simulink model "ConverterDesign_R2015a"  (R2015a)
settings: Solver=FixedStepDiscrete  SolverMode=SingleTasking  StartTime=0.0  StopTime=15  FixedStep=10e-6  RelTol=1e-3
undefined symbols (not defined in the file): Ion, Lithium
libraries: powerlib x13, simulink x2, powerlib_meascontrol x2, electricdrivelib x1, re_lib x1
settings Model: CovMetricSettings=dwe  CovHtmlReporting=off  covSaveCumulativeToWorkspaceVar=off  CovSaveSingleToWorkspaceVar=off  CovExternalEMLEnable=on  Creator=debma  LastModifiedBy=debma
settings DataIOCC: LimitDataPoints=off  SaveFormat=Dataset  ReturnWorkspaceOutputs=on
settings DebuggingCC: SFUnexpectedBacktrackingDiag=error  SFNoUnconditionalDefaultTransitionDiag=error
settings HardwareCC: ProdBitPerPointer=64  ProdLargestAtomicFloat=Float  ProdIntDivRoundTo=Zero  ProdEndianess=LittleEndian  ProdHWDeviceType=Specified
settings ModelReferenceCC: PropagateSignalLabelsOutOfModel=on
settings SFSimCC: SimUseLocalCustomCode=on
settings RTWCC: RTWUseLocalCustomCode=on
settings GRTTargetCC: TargetLangStandard=C99 (ISO)
settings ConfigurationSet: Description=Simscape Multibody

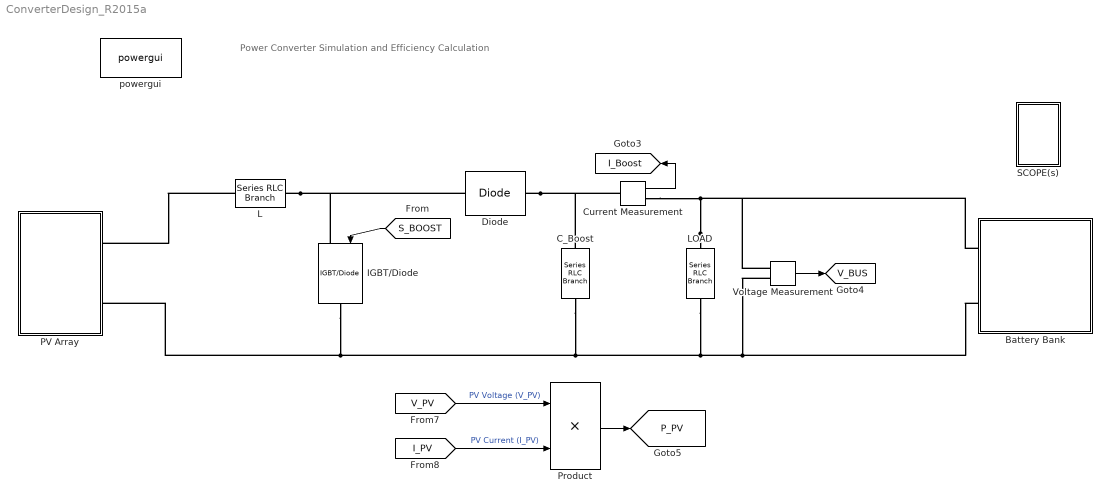
== system ConverterDesign_R2015a ==
  note: Power Converter Simulation and Efficiency Calculation
  Battery Bank : Subsystem
  C_Boost : powerlib/Elements/Series RLC Branch  LConnTagsString=__new0  RConnTagsString=__new0  BranchType=RC  Resistance=1e-4  Inductance=1e-3  SetiL0=off  InitialCurrent=0  Capacitance=3330e-6  Setx0=off  InitialVoltage=0  Measurements=None
  Current Measurement : powerlib/Measurements/Current Measurement  PhasorSimulation=off  OutputType=Complex  PSBequivalent=0
  Diode : powerlib/Power Electronics/Diode  Ron=0.001  Lon=0  Vf=0.8  IC=0  UseSnubber=0  Rs=500  Cs=250e-9  Measurements=off
  IGBT/Diode : powerlib/Power Electronics/IGBT//Diode  Ron=1e-3  Rs=1e5  Cs=inf  Measurements=off
  L : powerlib/Elements/Series RLC Branch  LConnTagsString=__new0  RConnTagsString=__new0  BranchType=RL  Resistance=0.1  Inductance=5e-3  SetiL0=off  InitialCurrent=0  Capacitance=100e-6  Setx0=off  InitialVoltage=0  Measurements=None
  LOAD : powerlib/Elements/Series RLC Branch  LConnTagsString=__new0  RConnTagsString=__new0  BranchType=R  Resistance=6  Inductance=1e-3  SetiL0=off  InitialCurrent=0  Capacitance=3330e-6  Setx0=off  InitialVoltage=0  Measurements=None
  PV Array : Subsystem
  Product : Product
  SCOPE(s) : Subsystem
  Voltage Measurement : powerlib/Measurements/Voltage Measurement  PhasorSimulation=off  OutputType=Complex  PSBequivalent=0
  powergui : powerlib/powergui  Priority=1  SimulationMode=Discrete  SampleTime=10e-6  frequency=60  Iterations=50  frequencyindice=0  Pbase=100e6  ErrMax=1e-4  UnitsV=kV  UnitsW=MW  buscounter=0  FunctionMessages=off  echomessages=off  EnableUseOfTLC=off  CurrentSourceSwitches=off  DisableSnubberDevices=off  DisableRonSwitches=off  DisableVfSwitches=off  DisplayEquations=off  AutomaticDiscreteSolvers=off  SolverType=Tustin/Backward Euler (TBE)  Interpol=off  ExternalGateDelay=off  methode=off  Ts=100  x0status=blocks  SPID=on  SwTol=0  HookPort=off  NonlinearTolerance=1e-4  nMaxIteration=100  ContinueOnMaxIteration=off  RestoreLinks=warning  ResistiveCurrentMeasurement=off  Frange=[0:2:500]  Ylog=off  Xlog=on  ShowGrid=off  save=off  variable=ZData  structure=0  ZoomFFT=off  StartTime=0.0  cycles=1  DisplayStyle=1  fundamental=60  FreqAxis=off  MaxFrequency=1000  frequencyindicesteady=1  RmsSteady=1  display=off
  tag scope: I_Boost=global, P_PV=global, V_BUS=global
  wires:
  Current Measurement/1 -> [I_Boost]
  Voltage Measurement/1 -> [V_BUS]
  [S_BOOST] -> IGBT/Diode/1
  Product/1 -> [P_PV]
  [I_PV] -> Product/2  "PV Current (I_PV)"
  [V_PV] -> Product/1  "PV Voltage (V_PV)"
  connections:
  Voltage Measurement/LConn2 -- Battery Bank/LConn2 -- LOAD/RConn1 -- C_Boost/RConn1 -- IGBT/Diode/RConn1 -- PV Array/RConn2
  Diode/RConn1 -- C_Boost/LConn1 -- Current Measurement/LConn1
  LOAD/LConn1 -- Voltage Measurement/LConn1 -- Battery Bank/LConn1 -- Current Measurement/RConn1
  L/RConn1 -- IGBT/Diode/LConn1 -- Diode/LConn1
  L/LConn1 -- PV Array/RConn1

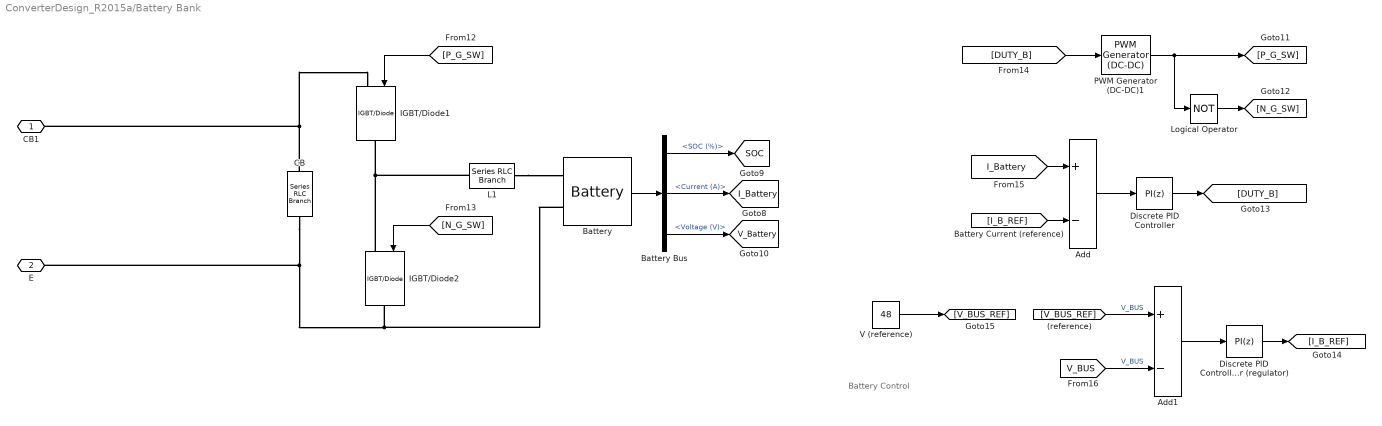
== system ConverterDesign_R2015a/Battery Bank ==
  note: Battery Control
  Add : Sum  Inputs=+-
  Add1 : Sum  Inputs=+-
  Battery : electricdrivelib/Extra Sources/Battery  BatType=Lithium-Ion  ShowTempParam=off  ThermalPreset=no  ShowAgeParam=off  NomV=24  NomQ=50  SOC=45  Batt_Tr=1  PresetModel=on  MaxQ=50  MinV=18  FullV=27.9357  Dis_rate=21.7391  R=0.0048  Normal_OP=45.2174  expZone="[25.9293      2.45652]"  current=[6.5 13 32.5]  Units=Time  Tci=20  NomT=20  T2=-30  MaxQ2=4.8  FullV2=7.1  Normal_OP2=5.655  expZone2="[6.58           1]"  Rca=0.6  ti=2000  Dp=0  Neq0=0  Tsim=1e6  Ta1=25  Qeol=5.4*0.9  Reol=0.013333*1.2  Char_age=[2.3478, 3]  Dis_age=[2.3478, 10]  N1=1500  N2=10500  N3=1000  N4=1400  Ta2=45  N5=950
  Battery Bus : BusSelector  OutputSignals=SOC (%),Current (A),Voltage (V)
  CB : powerlib/Elements/Series RLC Branch  LConnTagsString=__new0  RConnTagsString=__new0  BranchType=RC  Resistance=1e-4  Inductance=1e-3  SetiL0=off  InitialCurrent=0  Capacitance=1000e-6  Setx0=off  InitialVoltage=0  Measurements=None
  Discrete PID Controller : simulink/Continuous/PID Controller  Controller=PI  Form=Parallel  TimeDomain=Discrete-time  SampleTime=50e-6  IntegratorMethod=Forward Euler  FilterMethod=Forward Euler  ControllerParametersSource=internal  P=0.01  I=10  D=0  UseFilter=on  N=100  InitialConditionSource=internal  InitialConditionForIntegrator=0  InitialConditionForFilter=0  DifferentiatorICPrevScaledInput=0  ExternalReset=none  TrackingMode=off  Kt=1  LimitOutput=on  UpperSaturationLimit=0.95  LowerSaturationLimit=0  LinearizeAsGain=off  AntiWindupMode=none  Kb=1  POutMin=[]  POutMax=[]  IOutMin=[]  IOutMax=[]  DOutMin=[]  DOutMax=[]  NOutMin=[]  NOutMax=[]  SumOutMin=[]  SumOutMax=[]  SaturationOutMin=[]  SaturationOutMax=[]  PParamMin=[]  PParamMax=[]  IParamMin=[]  IParamMax=[]  DParamMin=[]  DParamMax=[]  NParamMin=[]  NParamMax=[]  KbParamMin=[]  KbParamMax=[]  KtParamMin=[]  KtParamMax=[]  KbOutMin=[]  KbOutMax=[]  KtOutMin=[]  KtOutMax=[]  IntegratorOutMin=[]  IntegratorOutMax=[]  FilterOutMin=[]  FilterOutMax=[]  SumI1OutMin=[]  SumI1OutMax=[]  SumI2OutMin=[]  SumI2OutMax=[]  SumI3OutMin=[]  SumI3OutMax=[]  SumDOutMin=[]  SumDOutMax=[]  DifferentiatorOutMin=[]  DifferentiatorOutMax=[]  IntegratorContinuousStateAttributes=''  IntegratorStateMustResolveToSignalObject=off  IntegratorRTWStateStorageClass=Auto  FilterContinuousStateAttributes=''  FilterStateMustResolveToSignalObject=off  FilterRTWStateStorageClass=Auto
  Discrete PID Controller (regulator) : simulink/Continuous/PID Controller  Controller=PI  Form=Parallel  TimeDomain=Discrete-time  SampleTime=500e-6  IntegratorMethod=Forward Euler  FilterMethod=Forward Euler  ControllerParametersSource=internal  P=0.85  I=10  D=0  UseFilter=on  N=100  InitialConditionSource=internal  InitialConditionForIntegrator=0  InitialConditionForFilter=0  DifferentiatorICPrevScaledInput=0  ExternalReset=none  TrackingMode=off  Kt=1  LimitOutput=on  UpperSaturationLimit=22  LowerSaturationLimit=-22  LinearizeAsGain=off  AntiWindupMode=none  Kb=1  POutMin=[]  POutMax=[]  IOutMin=[]  IOutMax=[]  DOutMin=[]  DOutMax=[]  NOutMin=[]  NOutMax=[]  SumOutMin=[]  SumOutMax=[]  SaturationOutMin=[]  SaturationOutMax=[]  PParamMin=[]  PParamMax=[]  IParamMin=[]  IParamMax=[]  DParamMin=[]  DParamMax=[]  NParamMin=[]  NParamMax=[]  KbParamMin=[]  KbParamMax=[]  KtParamMin=[]  KtParamMax=[]  KbOutMin=[]  KbOutMax=[]  KtOutMin=[]  KtOutMax=[]  IntegratorOutMin=[]  IntegratorOutMax=[]  FilterOutMin=[]  FilterOutMax=[]  SumI1OutMin=[]  SumI1OutMax=[]  SumI2OutMin=[]  SumI2OutMax=[]  SumI3OutMin=[]  SumI3OutMax=[]  SumDOutMin=[]  SumDOutMax=[]  DifferentiatorOutMin=[]  DifferentiatorOutMax=[]  IntegratorContinuousStateAttributes=''  IntegratorStateMustResolveToSignalObject=off  IntegratorRTWStateStorageClass=Auto  FilterContinuousStateAttributes=''  FilterStateMustResolveToSignalObject=off  FilterRTWStateStorageClass=Auto
  IGBT/Diode1 : powerlib/Power Electronics/IGBT//Diode  Ron=1e-3  Rs=1e5  Cs=inf  Measurements=off
  IGBT/Diode2 : powerlib/Power Electronics/IGBT//Diode  Ron=1e-3  Rs=1e5  Cs=inf  Measurements=off
  L1 : powerlib/Elements/Series RLC Branch  LConnTagsString=__new0  RConnTagsString=__new0  BranchType=RL  Resistance=0.1  Inductance=0.5e-3  SetiL0=off  InitialCurrent=0  Capacitance=100e-6  Setx0=off  InitialVoltage=0  Measurements=None
  Logical Operator : Logic  Operator=NOT  AllPortsSameDT=off  OutDataTypeStr=boolean
  PWM Generator (DC-DC)1 : powerlib_meascontrol/Pulse & Signal Generators/PWM Generator (DC-DC)  Fsw=5000  Ts=10e-6
  V (reference) : Constant  Value=48
  CB1 : PMIOPort  Side=Left
  E : PMIOPort  Port=2  Side=Left
  tag scope: I_Battery=global, SOC=global, V_Battery=global
  wires:
  Battery Bus/2 -> [I_Battery]  "<Current (A)>"
  Battery/1 -> Battery Bus/1
  Battery Bus/3 -> [V_Battery]  "<Voltage (V)>"
  [N_G_SW] -> IGBT/Diode2/1
  Battery Bus/1 -> [SOC]  "<SOC (%)>"
  [P_G_SW] -> IGBT/Diode1/1
  [I_B_REF] -> Add/2
  [I_Battery] -> Add/1
  [V_BUS] -> Add1/2  "V_BUS"
  Add/1 -> Discrete PID Controller/1
  [V_BUS_REF] -> Add1/1  "V_BUS"
  V (reference)/1 -> [V_BUS_REF]
  [DUTY_B] -> PWM Generator (DC-DC)1/1
  Logical Operator/1 -> [N_G_SW]
  PWM Generator (DC-DC)1/1 -> Logical Operator/1, [P_G_SW]
  Discrete PID Controller/1 -> [DUTY_B]
  Discrete PID Controller (regulator)/1 -> [I_B_REF]
  Add1/1 -> Discrete PID Controller (regulator)/1
  connections:
  L1/LConn1 -- IGBT/Diode2/LConn1 -- IGBT/Diode1/RConn1
  Battery/LConn2 -- CB/RConn1 -- E/RConn1 -- IGBT/Diode2/RConn1
  IGBT/Diode1/LConn1 -- CB/LConn1 -- CB1/RConn1
  L1/RConn1 -- Battery/LConn1

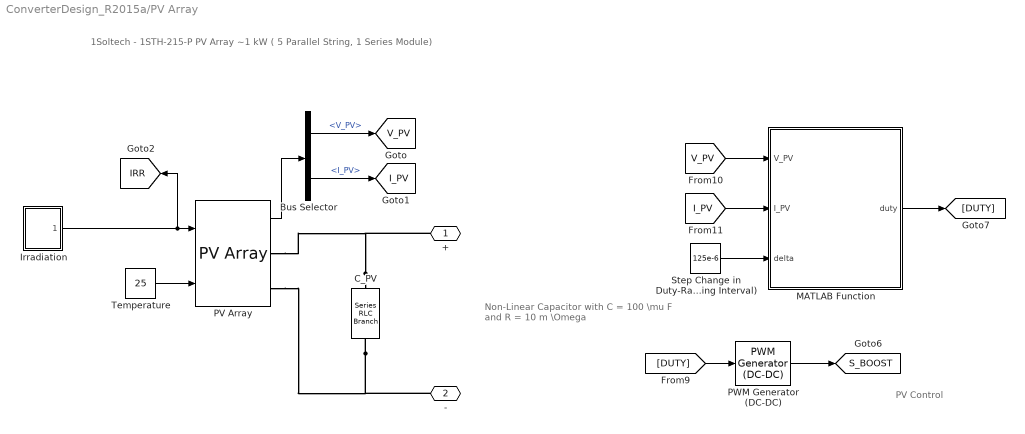
== system ConverterDesign_R2015a/PV Array ==
  note: Non-Linear Capacitor
      | with C = 100 \mu F and R = 10 m \Omega
  note: 1Soltech - 1STH-215-P PV Array
      | ~1 kW ( 5 Parallel String, 1 Series Module)
  note: PV Control
  Bus Selector : BusSelector  OutputSignals=V_PV,I_PV
  C_PV : powerlib/Elements/Series RLC Branch  LConnTagsString=__new0  RConnTagsString=__new0  BranchType=RC  Resistance=1e-3  Inductance=1e-3  SetiL0=off  InitialCurrent=0  Capacitance=100e-6  Setx0=off  InitialVoltage=0  Measurements=None
  Irradiation : Subsystem
  MATLAB Function : MATLAB Function  TreatAsAtomicUnit=on
      settings: PermitHierarchicalResolution=ParametersOnly
  PV Array : re_lib/Solar/PV Array  Npar=5  Nser=1  PlotType=array @ 1000 W/m2 & specified temperatures  S_vec="[ 1000  500  100 ]"  Temp_C_vec="[ 45 25  ]"  ModuleName=1Soltech 1STH-215-P  PlotWhenSelected=off  Pm=213.15  Ncell=60  Voc=36.3  Isc=7.84  Vm=29  Im=7.35  beta_Voc_pc=-0.36099  alpha_Isc_pc=0.102  beta_Voc=-0.13104  alpha_Isc=0.007997  IL=7.8649  I0=2.9259e-10  nI=0.98117  Rsh=313.3991  Rs=0.39383  RobustModel=off  RobustCellTemperature=25  BAL=on  Tc=1e-6  Tfilter=5e-5
  PWM Generator (DC-DC) : powerlib_meascontrol/Pulse & Signal Generators/PWM Generator (DC-DC)  Fsw=5000  Ts=10e-6
  Step Change in Duty-Ratio (for Each Sampling Interval) : Constant  Value=125e-6
  Temperature : Constant  Value=25
  + : PMIOPort  Side=Right
  - : PMIOPort  Port=2  Side=Right
  tag scope: IRR=global, I_PV=global, S_BOOST=global, V_PV=global
  wires:
  Bus Selector/1 -> [V_PV]  "<V_PV>"
  Bus Selector/2 -> [I_PV]  "<I_PV>"
  PV Array/1 -> Bus Selector/1
  Temperature/1 -> PV Array/2
  PWM Generator (DC-DC)/1 -> [S_BOOST]
  [DUTY] -> PWM Generator (DC-DC)/1
  Step Change in Duty-Ratio (for Each Sampling Interval)/1 -> MATLAB Function/3(delta)
  [V_PV] -> MATLAB Function/1(V_PV)
  [I_PV] -> MATLAB Function/2(I_PV)
  MATLAB Function/1(duty) -> [DUTY]
  Irradiation/1(Out1) -> [IRR], PV Array/1
  connections:
  C_PV/RConn1 -- PV Array/RConn2 -- -/RConn1
  C_PV/LConn1 -- +/RConn1 -- PV Array/RConn1

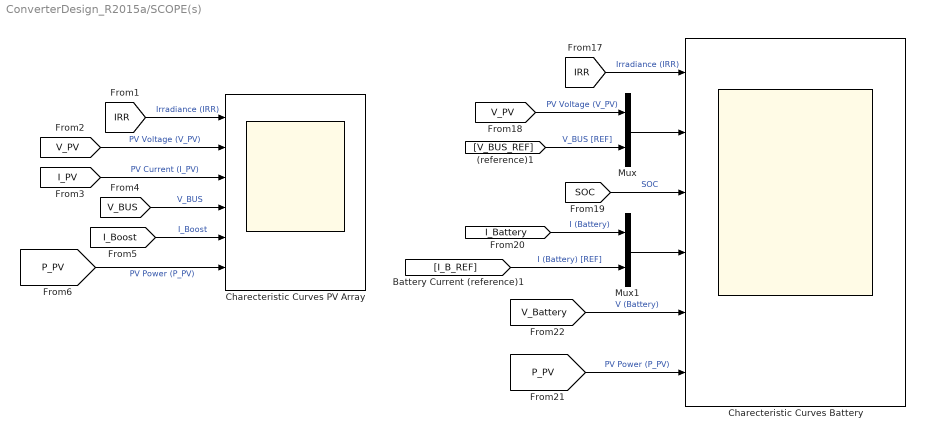
== system ConverterDesign_R2015a/SCOPE(s) ==
  Charecteristic Curves Battery : Scope  NumInputPorts=6
      settings: TimeRange=auto  TickLabels=on  ShowLegends=on  MaxDataPoints=5000  SaveToWorkspace=off  YMin=656.25~-3918227962833602784781855839214090586422740458343102423236608.00000~-5.625~-23185476129448355143547242404245563380754995478528.00000~-14794837847731686204552179595717563784263368704.00000~-12056188561590079438161559989034212797808582161761117921872976968295093132765543006049931381634112028085018214341355241472.00000  YMax=1593.75~457985303845118023392705621322677339993943161743665000349696.00000~50.625~208669285165035230041854762114589655875021099237376.00000~1643870871970187039148703231355712268520128512.00000~104063030908154254868941265509442788744971211883809997698507250318196589914636696782452885477526784590298016965099626954752.00000  SampleTime=-1
  Charecteristic Curves PV Array : Scope  NumInputPorts=6
      settings: TimeRange=auto  TickLabels=on  MaxDataPoints=5000  SaveToWorkspace=off  SaveName=ScopeData  YMin=656.25~-3918227962833602784781855839214090586422740458343102423236608.00000~-39255033157738301146592537600866684433175411425194587059126272.00000~-322637594827773546335669899078563623774149068980224.00000~-161406945548328037456087972305374274335800240596058112.00000~-12056188561590079438161559989034212797808582161761117921872976968295093132765543006049931381634112028085018214341355241472.00000  YMax=1593.75~457985303845118023392705621322677339993943161743665000349696.00000~4503493206297146506974009941854996624004127598499182627782656.00000~35848621647530383075781065212982075743857645977600.00000~17934105060925335427432892368505783742500155185692672.00000~104063030908154254868941265509442788744971211883809997698507250318196589914636696782452885477526784590298016965099626954752.00000  SampleTime=-1
  Mux : Mux  Inputs=2
  Mux1 : Mux  Inputs=2
  wires:
  [I_PV] -> Charecteristic Curves PV Array/3  "PV Current (I_PV)"
  [P_PV] -> Charecteristic Curves PV Array/6  "PV Power (P_PV)"
  Mux1/1 -> Charecteristic Curves Battery/4
  [V_PV] -> Charecteristic Curves PV Array/2  "PV Voltage (V_PV)"
  [V_BUS] -> Charecteristic Curves PV Array/4  "V_BUS"
  [I_B_REF] -> Mux1/2  "I (Battery) [REF]"
  [P_PV] -> Charecteristic Curves Battery/6  "PV Power (P_PV)"
  [I_Battery] -> Mux1/1  "I (Battery)"
  [V_Battery] -> Charecteristic Curves Battery/5  "V (Battery)"
  [IRR] -> Charecteristic Curves PV Array/1  "Irradiance (IRR)"
  [SOC] -> Charecteristic Curves Battery/3  "SOC"
  [I_Boost] -> Charecteristic Curves PV Array/5  "I_Boost"
  [V_BUS_REF] -> Mux/2  "V_BUS [REF]"
  [V_PV] -> Mux/1  "PV Voltage (V_PV)"
  [IRR] -> Charecteristic Curves Battery/1  "Irradiance (IRR)"
  Mux/1 -> Charecteristic Curves Battery/2

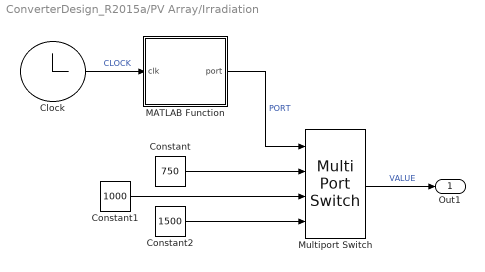
== system ConverterDesign_R2015a/PV Array/Irradiation ==
  Clock : Clock
  Constant : Constant  Value=750
  Constant1 : Constant  Value=1000
  Constant2 : Constant  Value=1500
  MATLAB Function : MATLAB Function  TreatAsAtomicUnit=on
      settings: PermitHierarchicalResolution=ParametersOnly
  Multiport Switch : MultiPortSwitch
  Out1 : Outport
  wires:
  Multiport Switch/1 -> Out1/1  "VALUE"
  Clock/1 -> MATLAB Function/1(clk)  "CLOCK"
  MATLAB Function/1(port) -> Multiport Switch/1  "PORT"
  Constant/1 -> Multiport Switch/2
  Constant1/1 -> Multiport Switch/3
  Constant2/1 -> Multiport Switch/4

== matlab function ConverterDesign_R2015a/PV Array/Irradiation/MATLAB Function ==
  data: clk input; port output
%% A Function to select different port of Multi-Port Switch
function port = PortSelection(clk)
    % Given the Simulation-Clock and Multi-Port Switch, with 3-Cases
    % this function divides the total simulation time into 3-interval
    % and based on it, activates the multi-port switch
    % uses the variable SIM_TIME
    % defined in Model Callbacks
    
    if clk <= 5
        port = 1;
    elseif clk > 5 && clk < 10
        port = 2;
    else
        port = 3;
    end

== matlab function ConverterDesign_R2015a/PV Array/MATLAB Function ==
  data: V_PV input; duty output; I_PV input; delta input
%% MPPT Algorithm, as given by Naki GÜLER in his Video
function duty = MPPT_Algorithm(V_PV, I_PV, delta)
    % First, define the initial Duty Ratio (D)
    D_INIT = 0.05;
    % A min & max D is defined
    D_MIN = 0;
    D_MAX = 0.75;
    
    persistent V_OLD P_OLD D_OLD; % defined, so that these variables,
    % can be accessed everytime, and the old value can be obtained by the
    % difference the old and the new value.
    if isempty(V_OLD)
        V_OLD = 0;
        P_OLD = 0;
        D_OLD = D_INIT;
    end
    
    P = V_PV * I_PV; % Calculated Power
    
    % Calculating delta values, for MPPT Algorithm
    dV = V_PV - V_OLD;
    dP = P - P_OLD;
    
    %% P&O Method of MPPT Tracking Algorithm
    if dP ~= 0 && V_PV > 30
        if dP < 0
            if dV < 0
                duty = D_OLD - delta;
            else
                duty = D_OLD + delta;
            end
        else
            if dV < 0
                duty = D_OLD + delta;
            else
                duty = D_OLD - delta;
            end
        end
    else
        duty = D_OLD;
    end
    
    if duty >= D_MAX
        duty = D_MAX;
    elseif duty < D_MIN
        duty = D_MIN;
    end
    
    %% Setting the OLD Values with the Current Condition Value
    D_OLD = duty;
    V_OLD = V_PV;
    P_OLD = P;
